simulink model "Dynamic_Vibration_Absorber"  (R2023b)
settings: Solver=VariableStepAuto  StartTime=0.0  StopTime=10  MaxStep=0.001  RelTol=1e-3
model workspace (MAT data in the model file):
  b = 100
  k1 = 100
  k2 = 400
  m1 = 20
  m2 = 200
settings Model: Creator=91839  LastModifiedBy=siva kumar
settings SolverCC: AlgebraicLoopSolver=TrustRegion
settings DataIOCC: ExternalInput=data  SaveFormat=Array  DSMLogging=off  ReturnWorkspaceOutputs=off
settings DebuggingCC: UnconnectedInputMsg=warning  UnconnectedOutputMsg=warning  UnconnectedLineMsg=warning
settings ModelReferenceCC: EnableRefExpFcnMdlSchedulingChecks=on
settings SFSimCC: CustomCodeUndefinedFunction=UseInterfaceOnly

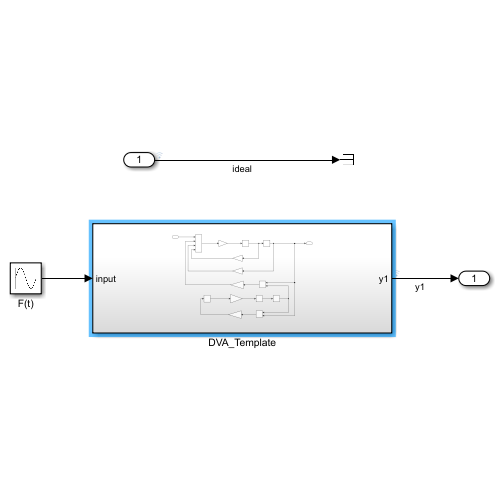
[thumbnail: Simulink's stored preview of the top-level diagram]
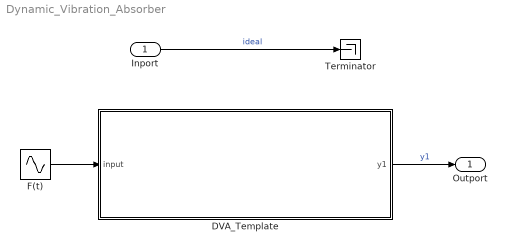
== system Dynamic_Vibration_Absorber ==
  Inport : Inport
  DVA_Template : Subsystem
  F(t) : Sin  Frequency=2  SampleTime=0
  Terminator : Terminator
  Outport : Outport
  wires:
  Inport/1 -> Terminator/1  "ideal"
  F(t)/1 -> DVA_Template/1(input)
  DVA_Template/1(y1) -> Outport/1  "y1"

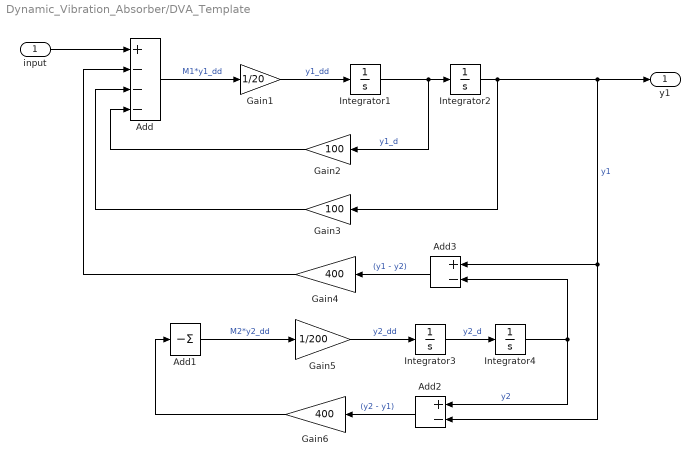
== system Dynamic_Vibration_Absorber/DVA_Template ==
  input : Inport
  Add : Sum  Inputs=+---
  Add1 : Sum  Inputs=-
  Add2 : Sum  Inputs=+-
  Add3 : Sum  Inputs=+-
  Gain1 : Gain  Gain=1/20
  Gain2 : Gain  Gain=100
  Gain3 : Gain  Gain=100
  Gain4 : Gain  Gain=400
  Gain5 : Gain  Gain=1/200
  Gain6 : Gain  Gain=400
  Integrator{1..4} (4 alike) : Integrator
  y1 : Outport
  wires:
  Add/1 -> Gain1/1  "M1*y1_dd"
  Gain1/1 -> Integrator1/1  "y1_dd"
  Integrator1/1 -> Integrator2/1, Gain2/1  "y1_d"
  Integrator2/1 -> y1/1, Add2/2, Add3/1, Gain3/1  "y1"
  Add1/1 -> Gain5/1  "M2*y2_dd"
  Integrator4/1 -> Add3/2, Add2/1  "y2"
  Integrator3/1 -> Integrator4/1  "y2_d"
  Gain5/1 -> Integrator3/1  "y2_dd"
  Add2/1 -> Gain6/1  "(y2 - y1)"
  Gain6/1 -> Add1/1
  Add3/1 -> Gain4/1  "(y1 - y2)"
  Gain4/1 -> Add/2
  input/1 -> Add/1
  Gain3/1 -> Add/3
  Gain2/1 -> Add/4
